simulink model "test"  (Simulink 5.0)
settings: Solver=FixedStepDiscrete  StartTime=0.0  StopTime=10.0  RelTol=1e-3
libraries: rtai_devices x1
settings Model: Creator=bucher  LastModifiedBy=bucher  ExtModeAutoUpdateStatusClock=off  RTWSystemTargetFile=rtai.tlc  RTWTemplateMakefile=rtai.tmf  RTWOptions="-aEnforceIntegerDowncast=1 -aFoldNonRolledExpr=1 -aForceParamTrailComments=0 -aGenerateComments=1 -aGenerateReport=0 -aIncDataTypeInIds=0 -aIncHierarchyInIds=0 -aInlineInvariantSignals=0 -aInlineParameters=0 -aInlinedPrmAccess=\"Literals\" -aLocalBlockOutputs=1 -aMaxRTWIdLen=31 -aPrefixModelToSubsysFcnNames=1 -aRTWVerbose=1 -aRollThreshold=5 -aShowEliminatedStatements=0"

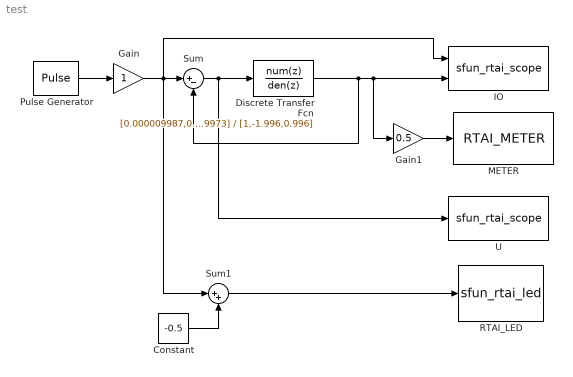
== system test ==
  Constant : Constant  Value=-0.5
  Discrete Transfer Fcn : DiscreteTransferFcn  Numerator=[0.000009987,0.000009973]  Denominator=[1,-1.996,0.996]  SampleTime=1e-3
  Gain : Gain  SaturateOnIntegerOverflow=on
  Gain1 : Gain  Gain=0.5  SaturateOnIntegerOverflow=on
  IO : S-Function  AncestorBlock=rtai_devices/RTAI_SCOPE  FunctionName=sfun_rtai_scope  Parameters=numch,ts  mask(RTAI SCOPE){numch=2, ts=-1}
      mask prompts: numch "Number of traces:"; ts "Sampling time [s] (-1 for inherited):"
      mask help: RTAI run-time scope
  METER : rtai_devices/RTAI_METER  dt=-1
  Pulse Generator : DiscretePulseGenerator  Period=10000  PulseWidth=5000  SampleTime=1e-3
  RTAI_LED : S-Function  AncestorBlock=rtai_devices/RTAI_LED  FunctionName=sfun_rtai_led  Parameters=n_leds,dt  mask(RTAI_LED){n_leds=1, dt=-1}
      mask prompts: n_leds "Number of leds (max 32) :"; dt "Sample time [s] (-1 for inherited) :"
      mask help: RTAI run time led
  Sum : Sum  Inputs=|+-  SaturateOnIntegerOverflow=on
  Sum1 : Sum  Inputs=|++  SaturateOnIntegerOverflow=on
  U : S-Function  AncestorBlock=rtai_devices/RTAI_SCOPE  FunctionName=sfun_rtai_scope  Parameters=numch,ts  mask(RTAI SCOPE){numch=1, ts=-1}
      mask prompts: numch "Number of traces:"; ts "Sampling time [s] (-1 for inherited):"
      mask help: RTAI run-time scope
  wires:
  Gain/1 -> Sum1/1, Sum/1, IO/1
  Sum/1 -> Discrete Transfer Fcn/1, U/1
  Discrete Transfer Fcn/1 -> Gain1/1, IO/2, Sum/2
  Constant/1 -> Sum1/2
  Pulse Generator/1 -> Gain/1
  Gain1/1 -> METER/1
  Sum1/1 -> RTAI_LED/1
